simulink model "Aplicatia_SC_4c"  (R2021b)
settings: Solver=VariableStepAuto  StartTime=0.0  StopTime=50  RelTol=1e-6
undefined symbols (not defined in the file): kbcv
settings Model: Creator=alexandra.szedlak-st  LastModifiedBy=alexandra.szedlak-st

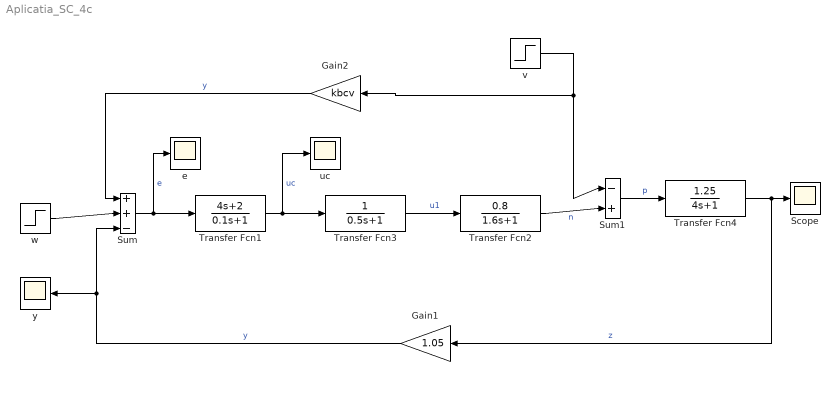
== system Aplicatia_SC_4c ==
  Gain1 : Gain  Gain=1.05
  Gain2 : Gain  Gain=kbcv
  Scope : Scope
  Sum : Sum  Inputs=|++-
  Sum1 : Sum  Inputs=|-+
  Transfer Fcn1 : TransferFcn  Numerator=[4 2]  Denominator=[0.1 1]
  Transfer Fcn2 : TransferFcn  Numerator=[0.8]  Denominator=[1.6 1]
  Transfer Fcn3 : TransferFcn  Denominator=[0.5 1]
  Transfer Fcn4 : TransferFcn  Numerator=[1.25]  Denominator=[4 1]
  e : Scope
  uc : Scope
  v : Step  Time=30  After=1.25  SampleTime=0
  w : Step  Time=0  After=7  SampleTime=0
  y : Scope
  wires:
  Transfer Fcn1/1 -> Transfer Fcn3/1, uc/1  "uc"
  Sum1/1 -> Transfer Fcn4/1  "p"
  Transfer Fcn2/1 -> Sum1/2  "n"
  Sum/1 -> Transfer Fcn1/1, e/1  "e"
  Transfer Fcn4/1 -> Gain1/1, Scope/1  "z"
  Gain1/1 -> Sum/3, y/1  "y"
  Transfer Fcn3/1 -> Transfer Fcn2/1  "u1"
  v/1 -> Gain2/1, Sum1/1
  w/1 -> Sum/2
  Gain2/1 -> Sum/1  "y"
